simulink library "tether001_ul"  (R2020a)
settings: Solver=VariableStepAuto  StartTime=0.0  StopTime=10.0  RelTol=1e-3
undefined symbols (not defined in the file or in its folder): f, fsolve, initNodePos, initNodeVel, numNodes, SampleTime, x0
libraries: nodePosToLinkPos_ul x1
settings Model: Creator=mitch  LastModifiedBy=mr-jo

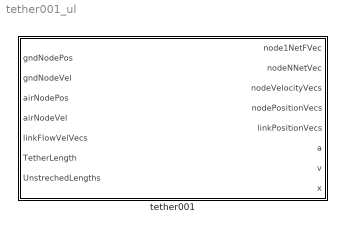
== system tether001_ul ==
  tether001 : Subsystem

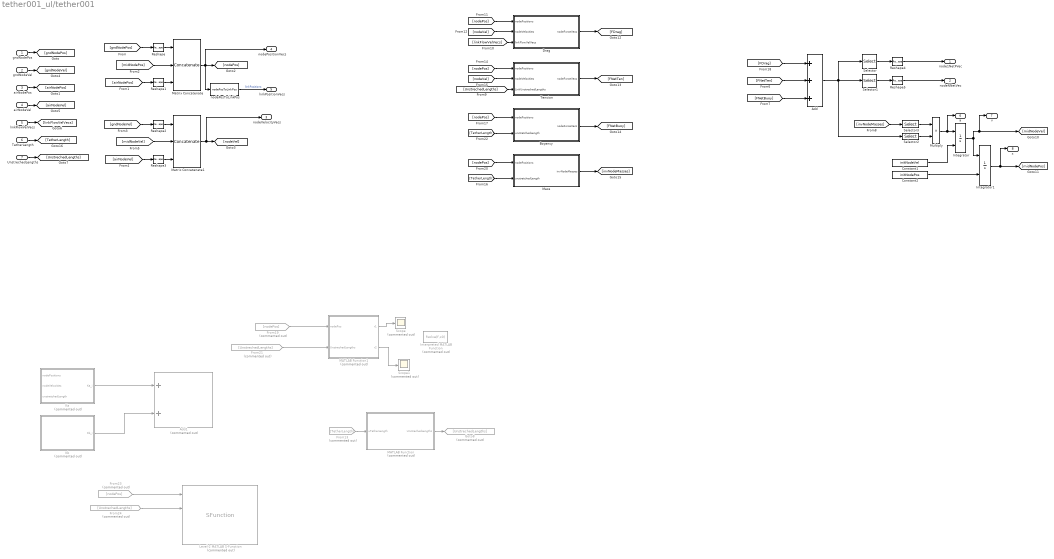
== system tether001_ul/tether001 ==
  gndNodePos : Inport
  gndNodeVel : Inport  Port=2
  airNodePos : Inport  Port=3
  airNodeVel : Inport  Port=4
  linkFlowVelVecs : Inport  Port=5
  TetherLength : Inport  Port=6
  UnstrechedLengths : Inport  Port=7
  Add : Sum  Inputs=3
  Add1 : Sum  Commented=on
  Boyancy : Subsystem
  Constant1 : Constant  Value=initNodeVel
  Constant2 : Constant  Value=initNodePos
  Drag : Subsystem
  From13 : From  Commented=on  GotoTag=TetherLength
  From19 : From  Commented=on  GotoTag=nodePos
  From21 : From  Commented=on  GotoTag=UnstrechedLengths
  From23 : From  Commented=on  GotoTag=nodePos
  From24 : From  Commented=on  GotoTag=UnstrechedLengths
  Goto8 : Goto  Commented=on  GotoTag=UnstrechedLengths
  Integrator : Integrator  InitialConditionSource=external
  Integrator1 : Integrator  InitialConditionSource=external
  Interpreted MATLAB Function : MATLABFcn  Commented=on  MATLABFcn=fsolve(f,x0)  Output1D=off
  Ka : MATLAB Function  Commented=on  TreatAsAtomicUnit=on
  Kb : MATLAB Function  Commented=on  TreatAsAtomicUnit=on
  Level-2 MATLAB S-Function : M-S-Function  Commented=on  FunctionName=SFunction
  MATLAB Function : MATLAB Function  Commented=on  TreatAsAtomicUnit=on
  MATLAB Function1 : MATLAB Function  Commented=on  TreatAsAtomicUnit=on
  Mass : Subsystem
  Matrix Concatenate : Concatenate  NumInputs=3  Mode=Multidimensional array  ConcatenateDimension=2
  Matrix Concatenate1 : Concatenate  NumInputs=3  Mode=Multidimensional array  ConcatenateDimension=2
  Multiply : Product
  Reshape{,1..5} (6 alike) : Reshape  OutputDimensionality=Column vector (2-D)
  Scope : Scope  Commented=on
  Scope1 : Scope  Commented=on
  Selector : Selector  NumberOfDimensions=2  InputPortWidth=3  IndexOptions=Select all,Index vector (dialog)  Indices=[1 3],1  OutputSizes=1,1
  Selector1 : Selector  NumberOfDimensions=2  InputPortWidth=3  IndexOptions=Select all,Index vector (dialog)  Indices=[1 3],1  OutputSizes=1,1
  Selector2 : Selector  NumberOfDimensions=2  InputPortWidth=3  IndexOptions=Select all,Index vector (dialog)  Indices=[1 3],2:numNodes-1  OutputSizes=1,1
  Selector3 : Selector  NumberOfDimensions=2  InputPortWidth=3  IndexOptions=Select all,Index vector (dialog)  Indices=[1 3],2:numNodes-1  OutputSizes=1,1
  Tension : Subsystem
  nodePosToLinkPos : nodePosToLinkPos_ul/nodePosToLinkPos  SystemSampleTime=-1  Latency=0  AutoFrameSizeCalculation=off
  node1NetFVec : Outport  SampleTime=SampleTime
  nodeNNetVec : Outport  Port=2  SampleTime=SampleTime
  nodeVelocityVecs : Outport  Port=3  SampleTime=SampleTime
  nodePositionVecs : Outport  Port=4  SampleTime=SampleTime
  linkPositionVecs : Outport  Port=5  SampleTime=SampleTime
  a : Outport  Port=6  SampleTime=SampleTime
  v : Outport  Port=7  SampleTime=SampleTime
  x : Outport  Port=8  SampleTime=SampleTime
  wires:
  Drag/1(nodeForceVecs) -> [FDrag]
  [FNetBuoy] -> Add/3
  [TetherLength] -> Boyancy/2(unstretchedLength)
  Reshape3/1 -> Matrix Concatenate1/3
  Reshape5/1 -> nodeNNetVec/1
  gndNodePos/1 -> [gndNodePos]
  [nodePos] -> Boyancy/1(nodePositions)
  Add/1 -> Selector2/1, Selector1/1, Selector/1
  Matrix Concatenate1/1 -> nodeVelocityVecs/1, [nodeVel]
  linkFlowVelVecs/1 -> [linkFlowVelVecs]
  Boyancy/1(nodeForceVecs) -> [FNetBuoy]
  Mass/1(invNodeMasses) -> [invNodeMasses]
  [linkFlowVelVecs] -> Drag/3(linkFlowVelVecs)
  Reshape4/1 -> node1NetFVec/1
  TetherLength/1 -> [TetherLength]
  [nodePos] -> Mass/1(nodePositions)
  [nodePos] -> Drag/1(nodePositions)
  [gndNodePos] -> Reshape/1
  [TetherLength] -> Mass/2(unstretchedLength)
  airNodeVel/1 -> [airNodeVel]
  Tension/1("nodeForceVecs ") -> [FNetTen]
  [nodeVel] -> Tension/2(nodeVelocities)
  [nodePos] -> Tension/1(nodePositions)
  [gndNodeVel] -> Reshape2/1
  Selector/1 -> Reshape4/1
  [airNodeVel] -> Reshape3/1
  [FDrag] -> Add/1
  Selector3/1 -> Multiply/1
  gndNodeVel/1 -> [gndNodeVel]
  [nodeVel] -> Drag/2(nodeVelocities)
  nodePosToLinkPos/1 -> linkPositionVecs/1  "linkPositions"
  Selector2/1 -> Multiply/2
  [FNetTen] -> Add/2
  Reshape2/1 -> Matrix Concatenate1/1
  Matrix Concatenate/1 -> nodePosToLinkPos/1, nodePositionVecs/1, [nodePos]
  [midNodePos] -> Matrix Concatenate/2
  [midNodeVel] -> Matrix Concatenate1/2
  [invNodeMasses] -> Selector3/1
  Reshape1/1 -> Matrix Concatenate/3
  Selector1/1 -> Reshape5/1
  airNodePos/1 -> [airNodePos]
  [airNodePos] -> Reshape1/1
  Reshape/1 -> Matrix Concatenate/1
  Constant1/1 -> Integrator/2
  Multiply/1 -> a/1, Integrator/1
  Constant2/1 -> Integrator1/2
  Integrator1/1 -> x/1, [midNodePos]
  Integrator/1 -> Integrator1/1, v/1, [midNodeVel]
  UnstrechedLengths/1 -> [UnstrechedLengths]
  [UnstrechedLengths] -> Tension/3(LinkUnstrechedLengths)
  From13/1 -> MATLAB Function/1(uTetherLength)
  MATLAB Function/1(UnstrechedLengths) -> Goto8/1
  Ka/1(Ka_i) -> Add1/1
  Kb/1(Kb_i) -> Add1/2
  From21/1 -> MATLAB Function1/2(UnstrechedLengths)
  From19/1 -> MATLAB Function1/1(nodePos)
  MATLAB Function1/1(r1) -> Scope/1
  MATLAB Function1/2(r2) -> Scope1/1
  From24/1 -> Level-2 MATLAB S-Function/2
  From23/1 -> Level-2 MATLAB S-Function/1

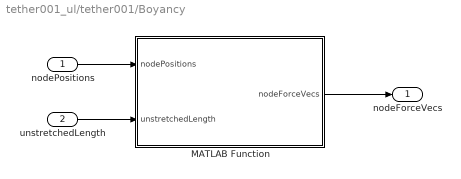
== system tether001_ul/tether001/Boyancy ==
  nodePositions : Inport
  unstretchedLength : Inport  Port=2
  MATLAB Function : MATLAB Function  TreatAsAtomicUnit=on
  nodeForceVecs : Outport  VectorParamsAs1DForOutWhenUnconnected=off
  wires:
  MATLAB Function/1(nodeForceVecs) -> nodeForceVecs/1
  unstretchedLength/1 -> MATLAB Function/2(unstretchedLength)
  nodePositions/1 -> MATLAB Function/1(nodePositions)

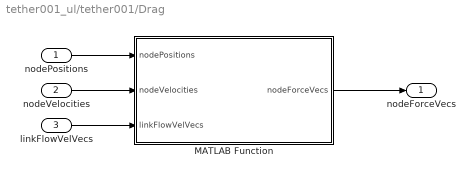
== system tether001_ul/tether001/Drag ==
  nodePositions : Inport
  nodeVelocities : Inport  Port=2
  linkFlowVelVecs : Inport  Port=3
  MATLAB Function : MATLAB Function  TreatAsAtomicUnit=on
  nodeForceVecs : Outport
  wires:
  nodePositions/1 -> MATLAB Function/1(nodePositions)
  linkFlowVelVecs/1 -> MATLAB Function/3(linkFlowVelVecs)
  MATLAB Function/1(nodeForceVecs) -> nodeForceVecs/1
  nodeVelocities/1 -> MATLAB Function/2(nodeVelocities)

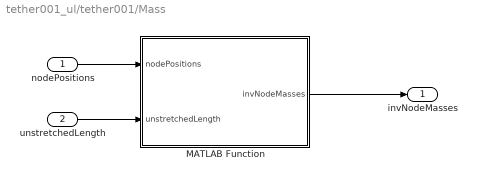
== system tether001_ul/tether001/Mass ==
  nodePositions : Inport
  unstretchedLength : Inport  Port=2
  MATLAB Function : MATLAB Function  TreatAsAtomicUnit=on
  invNodeMasses : Outport  VectorParamsAs1DForOutWhenUnconnected=off
  wires:
  nodePositions/1 -> MATLAB Function/1(nodePositions)
  unstretchedLength/1 -> MATLAB Function/2(unstretchedLength)
  MATLAB Function/1(invNodeMasses) -> invNodeMasses/1

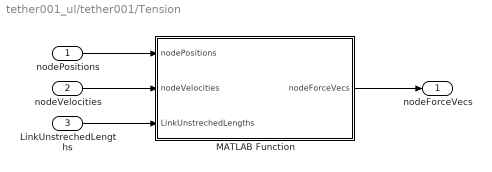
== system tether001_ul/tether001/Tension ==
  nodePositions : Inport
  nodeVelocities : Inport  Port=2
  LinkUnstrechedLengths : Inport  Port=3
  MATLAB Function : MATLAB Function  TreatAsAtomicUnit=on
  "nodeForceVecs " : Outport  VectorParamsAs1DForOutWhenUnconnected=off
  wires:
  nodeVelocities/1 -> MATLAB Function/2(nodeVelocities)
  LinkUnstrechedLengths/1 -> MATLAB Function/3(LinkUnstrechedLengths)
  nodePositions/1 -> MATLAB Function/1(nodePositions)
  MATLAB Function/1(nodeForceVecs) -> "nodeForceVecs "/1

== matlab function tether001_ul/tether001/Tension/MATLAB Function ==
  data: nodePositions input; nodeForceVecs output; nodeVelocities input; LinkUnstrechedLengths input
function nodeForceVecs = fcn(nodePositions, nodeVelocities, LinkUnstrechedLengths)
% clc
% clear
% nodePositions = [0,65,131,196,261,326,391,401;...
%                  0,0 ,0  ,0  ,0  ,0  ,0  ,0  ;...
%                  0,0 ,0  ,0  ,0  ,0  ,0  ,0  ];%linspace(0,TetherLength,numNodes)
% unstretchedLength = 400;
% LinkUnstrechedLengths = [65,65,65,65,65,65,10];
% nodeVelocities = zeros(3,8);

mass = .1;
zeta = .2;
diameter = .1;
youngsMod = 25000000000;

% Number of nodes
N = size(nodePositions,2);

% Spring constant and damping coefficient for each link
SpringConsts = youngsMod*(pi/4)*(diameter^2)./LinkUnstrechedLengths;
DampCoeffs = zeta*2*sqrt(SpringConsts*mass);

% Vector from one node to another
linkVecs  = diff(nodePositions,1,2);

% Length of each link
linkLength = sqrt(sum(linkVecs.^2));

% Link direction unit vectors
linkUnitVecs = linkVecs./repmat(sqrt(sum(linkVecs.^2,1)),[3 1]);

% Rate of change of vector from one node to another
linkLengthDeriv = dot(nodeVelocities(:,2:end)-nodeVelocities(:,1:end-1),linkUnitVecs);


% Magnitude of sprint force and damping force on each link
springForces = zeros(size(linkLength));
damperForces  = zeros(size(linkLengthDeriv));
for i = 1:N-1
    if linkLength(i)>LinkUnstrechedLengths(i)
        springForces(i) = SpringConsts(i)*(linkLength(i)-LinkUnstrechedLengths(i));
        damperForces(i) = DampCoeffs(i)*linkLengthDeriv(i);
    end
end

% Total force in each link
totalLinkForceVec = repmat(springForces+damperForces,[3 1]).*linkUnitVecs;

% Force on each node
nodeForceVecs = [totalLinkForceVec(:,1) diff(totalLinkForceVec,1,2) -totalLinkForceVec(:,end)];

end

== matlab function tether001_ul/tether001/Drag/MATLAB Function ==
  data: nodePositions input; nodeForceVecs output; nodeVelocities input; linkFlowVelVecs input
function nodeForceVecs = fcn(nodePositions, nodeVelocities, linkFlowVelVecs)

thrDiam = .1;
flowDensity = 1000;
dragCoeff = .5;
% In the notation here, N is the number of nodes, therefore you have N-1
% links between the nodes.

% Velocity and center of links 3xN-1
linkVelocities = (nodeVelocities(:,1:end-1) + nodeVelocities(:,2:end))/2;

% Apparent flow at center of links 3xN-1
linkAppFlow = linkFlowVelVecs - linkVelocities; %repmat(flowVel(:),[1 size(linkVelocities,2)]) - linkVelocities;
% linkAppFlow(3,:) = 0; % Origional model zeroed z component

% Link center apparent flow magnitude 3xN-1
linkAppFlowMag = sqrt(sum(linkAppFlow.^2)); % Sum over columns

% Normalize columns to get unit vector 3xN-1
dragDirUnitVec = linkAppFlow./repmat(linkAppFlowMag,[3 1]);

% If linkAppFlowMag is zero, dragDirUnitVec will have nans, patch to fix
% that with zeros
% dragDirUnitVec(:,linkAppFlowMag==0) = zeros(3,numel(linkAppFlowMag==0));

% Dynamic pressures at link centers 1xN-1
dynPress = 0.5*flowDensity*linkAppFlowMag.^2;

% Link lengths, diff over columns 1xN-1
linkLengths = sqrt(sum(diff(nodePositions,1,2).^2));

% Unit vectors in the direction of the link 3xN-1
linkUnitVecs = diff(nodePositions,1,2)./repmat(linkLengths,[3 1]);

% Projected areas of each link
projArea = thrDiam*linkLengths.*sqrt(sum(cross(linkUnitVecs,dragDirUnitVec).^2,1));

% Drag force on links
linkForceVecs = repmat(dragCoeff*dynPress.*projArea,[3 1]).*dragDirUnitVec;

% Drag force on nodes
nodeForceVecs = [linkForceVecs(:,1) (linkForceVecs(:,1:end-1)+linkForceVecs(:,2:end)) linkForceVecs(:,end)]/2;

end

== matlab function tether001_ul/tether001/Boyancy/MATLAB Function ==
  data: nodePositions input; nodeForceVecs output; unstretchedLength input
function nodeForceVecs = fcn(nodePositions, unstretchedLength)

tetherDensity = 915;
fluidDensity = 1000;
diameter = .1;
gravity = 9.81;

% In this notation, N is the number of nodes

% Length of each link 1xN-1
linkLengths = sqrt(sum(diff(nodePositions,1,2).^2));

% Total length of all links, assuming they're straight lines, scalar
numericalTotalLength = sum(linkLengths);

% Number of links, scalar
numLinks = size(linkLengths,2);

% Total volume based on unspooled length, scalar
analyticalTotalVol  = unstretchedLength*(pi/4)*diameter^2;

% Total mass, based on unspooled length, scalar
analyticalTotalMass = tetherDensity*analyticalTotalVol;

% Mass of each link, 1xN-1
linkMasses  = analyticalTotalMass*(linkLengths./numericalTotalLength);

% Volume of each link, 1xN-1
linkVolumes = analyticalTotalVol*(linkLengths./numericalTotalLength);

% Net force on the links (buoyancy - gravity) on each link, 3xN-1
linkNetForceVecs = [repmat([0 0]',[1 numLinks]);(-gravity*linkMasses + gravity*fluidDensity*linkVolumes)];

% Net force on the nodes, 3xN
nodeForceVecs = [linkNetForceVecs(:,1) linkNetForceVecs(:,1:end-1)+linkNetForceVecs(:,2:end) linkNetForceVecs(:,end)]/2;


end

== matlab function tether001_ul/tether001/Mass/MATLAB Function ==
  data: nodePositions input; invNodeMasses output; unstretchedLength input
function invNodeMasses = fcn(nodePositions, unstretchedLength)
% clc
% clear
%  nodePositions = [0,65,131,196,261,326,391,401;...
%                  0,0 ,0  ,0  ,0  ,0  ,0  ,0  ;...
%                  0,0 ,0  ,0  ,0  ,0  ,0  ,0  ];%linspace(0,TetherLength,numNodes)
% unstretchedLength = 400;
% LinkUnstrechedLengths = [65,65,65,65,65,65,10];
% nodeVelocities = zeros(3,8);

tetherDensity = 915;
diameter = .1;

% In this notation, N is the number of nodes

% Length of each link 1xN-1
linkLengths = sqrt(sum(diff(nodePositions,1,2).^2));

% Total length of all links, assuming they're straight lines, scalar
numericalTotalLength = sum(linkLengths);

% Total volume based on unspooled length, scalar
analyticalTotalVol  = unstretchedLength*(pi/4)*diameter^2;

% Total mass, based on unspooled length, scalar
analyticalTotalMass = tetherDensity*analyticalTotalVol;

% Mass of each link, 1xN-1
linkMasses  = analyticalTotalMass*(linkLengths./numericalTotalLength);

% 1/mass for each node, 3xN (repmat so that we can multiply with force
% vectors concatenated into matrix later
invNodeMasses = repmat(1./([linkMasses(1) linkMasses(1:end-1)+linkMasses(2:end) linkMasses(end)]/2),[3 1]);

end

== matlab function tether001_ul/tether001/Kb ==
  data: Kb_i output
function Kb_i = fcn()

N  = numNodes;
E  = 1;
I  = 1;
Li = 1;

Kb_i = ((E*I)/Li)*[zeros(N), eye(N) ,zeros(N),-eye(N) ;...
                   zeros(N),zeros(N),zeros(N),zeros(N);...
                   zeros(N),-eye(N) ,zeros(N), eye(N) ;...
                   zeros(N),zeros(N),zeros(N),zeros(N)];
end

== matlab function tether001_ul/tether001/Ka ==
  data: Ka_i output; nodePositions input; nodeVelocities input; unstretchedLength input
function Ka_i = fcn(nodePositions, nodeVelocities, unstretchedLength)
%function Ka_i = fcn(nodePositions, nodeVelocities, unstretchedLength)
clc
clear
NumNodes = 6;
%function Ka_i = fcn(nodePositions, nodeVelocities, unstretchedLength)
nodePositions = [0,1,2,3,4,10;0,1,2,3,4,5;0,1,2,3,4,5];
nodeVelocities = ones(3,NumNodes);

mass = .1;
zeta = .2;
diameter = .1;
youngsMod = 25000000000;

% Number of nodes
N = size(nodePositions,2);

% Spring constant and damping coefficient for each link
SpringConsts = youngsMod*(pi/4)*(diameter^2)./LinkUnstrechedLengths;
DampCoeffs = zeta*2*sqrt(SpringConsts*mass);

% Vector from one node to another
linkVecs  = diff(nodePositions,1,2);

% Length of each link
linkLength = sqrt(sum(linkVecs.^2));

% Link direction unit vectors
linkUnitVecs = linkVecs./repmat(sqrt(sum(linkVecs.^2,1)),[3 1]);

% Rate of change of vector from one node to another
linkLengthDeriv = dot(nodeVelocities(:,2:end)-nodeVelocities(:,1:end-1),linkUnitVecs);


% Magnitude of sprint force and damping force on each link
springForces = zeros(size(linkLength));
damperForces  = zeros(size(linkLengthDeriv));
for i = 1:N-1
    if linkLength(i)>LinkUnstrechedLengths(i)
        springForces(i) = SpringConsts(i)*(linkLength(i)-LinkUnstrechedLengths(i));
        damperForces(i) = DampCoeffs(i)*linkLengthDeriv(i);
    end
end

% Total force in each link
totalLinkForceVec = repmat(springForces+damperForces,[3 1]).*linkUnitVecs;

% Force on each node
nodeForceVecs = [totalLinkForceVec(:,1) diff(totalLinkForceVec,1,2) -totalLinkForceVec(:,end)];

li = 1;%unstrechedlength(i);
lami = (nodeForceVec-E*I*curvaturei^2);
Ka_i = [-(lami/Li)*eye(3) ,zeros(3)                  ,(lami/Li)*eye(3)  ,zeros(3)                  ;...
        zeros(3)          ,-(lami/45)*(Li^3)*eye(3)  ,zeros(3)          ,-(7*lami/360)*Li^3*eye(N) ;...
        (lami/Li)*eye(3)  ,zeros(3)                  ,-(lami/Li)*eye(3) ,zeros(3)                  ;...
        zeros(3)          ,-(7*lami/360)*Li^3*eye(N) ,zeros(3)          ,(lami/45)*(Li^3)*eye(3)   ];

== matlab function tether001_ul/tether001/MATLAB Function ==
  data: uTetherLength input; UnstrechedLengths output
function UnstrechedLengths = fcn(uTetherLength)
    UnstrechedLengths(1,:) = [((TetherLength(1)-LastLinkLength)/(numNodes-2))*ones(1,numNodes-2),LastLinkLength];
end

== matlab function tether001_ul/tether001/MATLAB Function1 ==
  data: r1 output; r2 output; nodePos input; UnstrechedLengths input
function [r1, r2] = fcn(nodePos, UnstrechedLengths)
%function [r1,r2] = fcn(nodePos,UnstrechedLengths)

% N = numNodes;
% L = UnstrechedLengths';
% r = nodePos;
N=6;
r = [0,1,2,3,4,5,6;...
     0,0,0,0,0,0,0;...
     0,0,0,0,0,0,0];
L = [1,1,1,1,1];

LUSE = [0,L,0];
Curvature_IC_mat1 = zeros(3*(N));
for i = 4:3:3*(N+1)
    for j = 4:3:3*(N+1)
        if i==j
            Curvature_IC_mat1((i-3):i-1,(j-3):(j-1)) = ((LUSE(((i-1)/3+1))+LUSE(((i-4)/3+1)))/3)*eye(3);
        elseif i==(j-3)
            Curvature_IC_mat1((i-3):i-1,(j-3):(j-1)) = ((LUSE(((i-1)/3+1)))/6)*eye(3);                
        elseif j==(i-3)
            Curvature_IC_mat1((i-3):i-1,(j-3):(j-1)) = ((LUSE(((i-4)/3+1)))/6)*eye(3);                
        end
    end
end

Curvature_IC_mat3 = zeros(3*(N),1);
Curvature_IC_mat3(1:3,1) = (r(:,2)-r(:,1))/LUSE(2);
for i = 7:3:3*(N)
    Curvature_IC_mat3(i-3:i-1) = (r(:,(i-1)/3+1)-r(:,(i-4)/3+1))/LUSE((i-1)/3+1)-(r(:,(i-4)/3+1)-r(:,(i-7)/3+1))/LUSE((i-4)/3+1);
end
Curvature_IC_mat3((end-2):end,1) = -(r(:,end)-r(:,(end-1)))/LUSE(end-1);
   

x0  = zeros(3*N,1);
f   = @(x)nonlinearsolver(x,Curvature_IC_mat1,Curvature_IC_mat3,N);
SOL = fsolve(f,x0); 

r1 = zeros(6,1);
for i = 1:6
    r1(i) = SOL(i);
end

r2 = zeros(3*(N-2),1);
for i = 7:length(SOL)
    r2(i-6) = SOL(i);
end

%end
